simulink model "MISSILE_SIM_3DANIM"  (R2020b)
settings: Solver=ode4  StartTime=0.0  StopTime=45  FixedStep=0.01  RelTol=1e-3  EnableMultiTasking=on
undefined symbols (not defined in the file): d2r, Ka, Kdc, Ki, Kr, l_T0, V_T, X_M0, X_T0, Z_M0, Z_T0
libraries: vrlib x3, simulink x1
settings Model: Creator=vinay  LastModifiedBy=LeChinh
settings DataIOCC: LimitDataPoints=on  SaveFormat=Array  ReturnWorkspaceOutputs=off
settings OptimizationCC: LifeSpan=inf
settings DebuggingCC: SFUnexpectedBacktrackingDiag=warning  SFNoUnconditionalDefaultTransitionDiag=warning  SFExecutionAtInitializationDiag=none  ArithmeticOperatorsInVariantConditions=warning
settings HardwareCC: ProdBitPerPointer=32  ProdBitPerSizeT=32  ProdBitPerPtrDiffT=32  ProdLargestAtomicFloat=None  ProdIntDivRoundTo=Undefined  ProdEndianess=Unspecified  ProdWordSize=32  ProdHWDeviceType=32-bit Generic
settings ModelReferenceCC: PropagateSignalLabelsOutOfModel=off
settings SFSimCC: SimUseLocalCustomCode=off  CustomCodeUndefinedFunction=UseInterfaceOnly
settings RTWCC: RTWUseLocalCustomCode=off
settings CodeAppCC: StateflowObjectComments=on
settings GRTTargetCC: TargetLangStandard=C89/C90 (ANSI)
settings ConfigComp: CovMetricSettings=dw  CovSaveCumulativeToWorkspaceVar=on  CovSaveSingleToWorkspaceVar=on  CovExternalEMLEnable=off

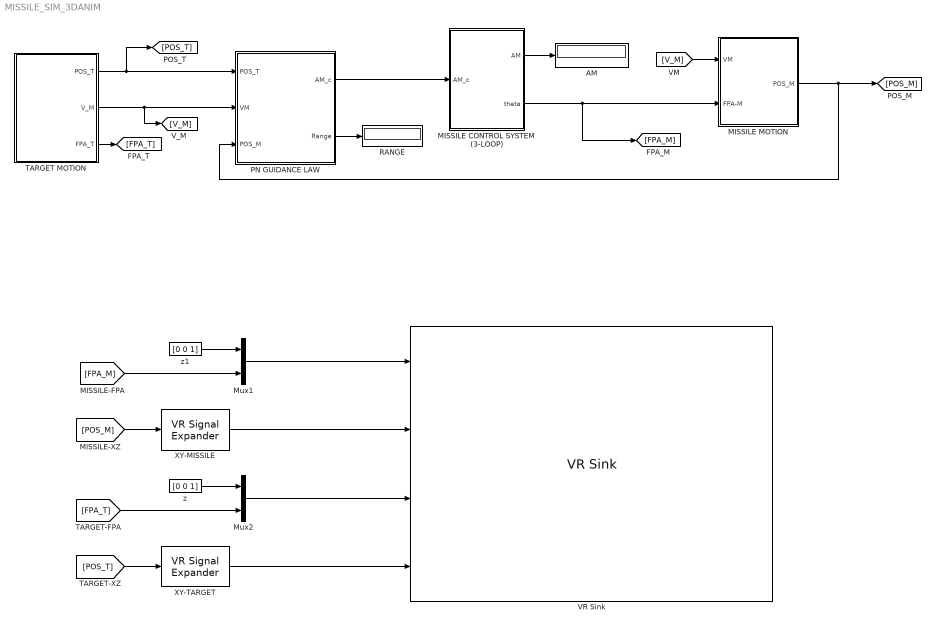
== system MISSILE_SIM_3DANIM ==
  AM : Display
  MISSILE CONTROL SYSTEM (3-LOOP) : Subsystem
  MISSILE MOTION : Subsystem
  Mux1 : Mux  Inputs=2
  Mux2 : Mux  Inputs=2
  PN GUIDANCE LAW : Subsystem
  RANGE : Display
  TARGET MOTION : Subsystem
  VR Sink : vrlib/VR Sink  InstantiateOnLoad=on  SampleTime=0.01  ViewEnable=on  RemoteChange=off  RemoteView=off  FieldsWritten=MISSILE-1_Scale.rotation.4.1.1.double#MISSILE-1_Scale.translation.3.1.1.double#UCAV_Halcyon_Test-3_Scale.rotation.4.1.1.double#UCAV_Halcyon_Test-3_Scale.translation.3.1.1.double  WorldFileName=interceptor_assembly.wrl  AutoView=off  VideoDimensions=[]  AllowVariableSize=off
  XY-MISSILE : vrlib/VR Signal Expander  outwidth=3  outidx=[1 2]
  XY-TARGET : vrlib/VR Signal Expander  outwidth=3  outidx=[1 2]
  z : Constant  Value=[0 0 1]
  z1 : Constant  Value=[0 0 1]
  wires:
  TARGET MOTION/1(POS_T) -> [POS_T], PN GUIDANCE LAW/1(POS_T)
  TARGET MOTION/2(V_M) -> [V_M], PN GUIDANCE LAW/2(VM)
  MISSILE MOTION/1(POS_M) -> PN GUIDANCE LAW/3(POS_M), [POS_M]
  MISSILE CONTROL SYSTEM (3-LOOP)/2(theta) -> [FPA_M], MISSILE MOTION/2(FPA-M)
  PN GUIDANCE LAW/1(AM_c) -> MISSILE CONTROL SYSTEM (3-LOOP)/1(AM_c)
  MISSILE CONTROL SYSTEM (3-LOOP)/1(AM) -> AM/1
  [V_M] -> MISSILE MOTION/1(VM)
  PN GUIDANCE LAW/2(Range) -> RANGE/1
  TARGET MOTION/3(FPA_T) -> [FPA_T]
  [POS_T] -> XY-TARGET/1
  [POS_M] -> XY-MISSILE/1
  [FPA_M] -> Mux1/2
  [FPA_T] -> Mux2/2
  z1/1 -> Mux1/1
  z/1 -> Mux2/1
  XY-MISSILE/1 -> VR Sink/2
  Mux2/1 -> VR Sink/3
  Mux1/1 -> VR Sink/1
  XY-TARGET/1 -> VR Sink/4

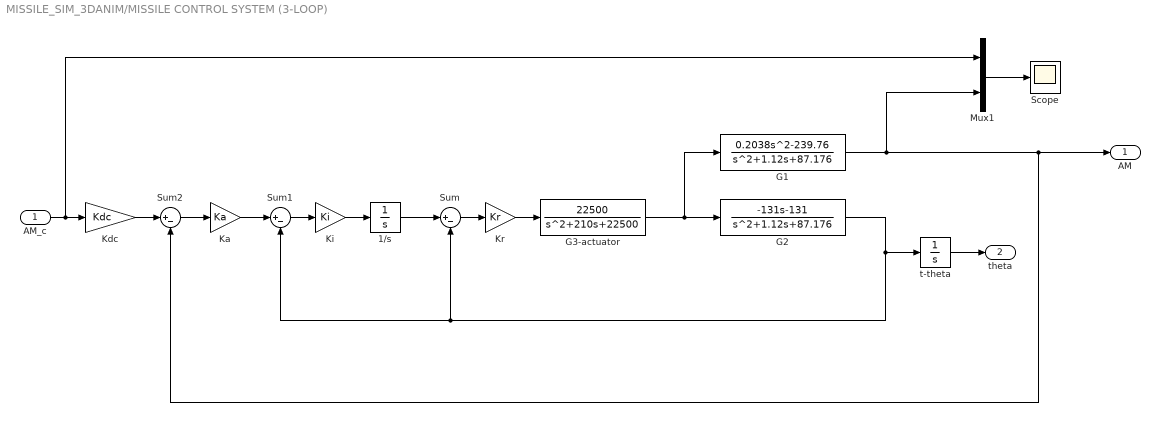
== system MISSILE_SIM_3DANIM/MISSILE CONTROL SYSTEM (3-LOOP) ==
  AM_c : Inport
  1/s : Integrator
  G1 : TransferFcn  Numerator=[0.2038, 0, -239.76]  Denominator=[1, 1.12, 87.176]
  G2 : TransferFcn  Numerator=[-131, -131]  Denominator=[1, 1.12, 87.176]
  G3-actuator : TransferFcn  Numerator=[22500]  Denominator=[1, 210, 22500]
  Ka : Gain  Gain=Ka
  Kdc : Gain  Gain=Kdc
  Ki : Gain  Gain=Ki
  Kr : Gain  Gain=Kr
  Mux1 : Mux  Inputs=2
  Scope : Scope
  Sum : Sum  Inputs=|+-
  Sum1 : Sum  Inputs=|+-
  Sum2 : Sum  Inputs=|+-
  t-theta : Integrator  InitialCondition=80*d2r
  AM : Outport
  theta : Outport  Port=2
  wires:
  Ki/1 -> 1/s/1
  Sum1/1 -> Ki/1
  t-theta/1 -> theta/1
  G3-actuator/1 -> G1/1, G2/1
  Kr/1 -> G3-actuator/1
  G2/1 -> t-theta/1, Sum1/2, Sum/2
  Sum/1 -> Kr/1
  1/s/1 -> Sum/1
  Ka/1 -> Sum1/1
  Kdc/1 -> Sum2/1
  Sum2/1 -> Ka/1
  AM_c/1 -> Mux1/1, Kdc/1
  G1/1 -> AM/1, Sum2/2, Mux1/2
  Mux1/1 -> Scope/1

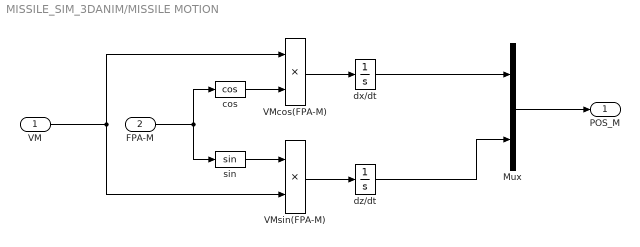
== system MISSILE_SIM_3DANIM/MISSILE MOTION ==
  VM : Inport
  FPA-M : Inport  Port=2
  Mux : Mux  Inputs=2
  VMcos(FPA-M) : Product
  VMsin(FPA-M) : Product
  cos : Trigonometry  Operator=cos
  dx/dt : Integrator  InitialCondition=X_M0
  dz/dt : Integrator  InitialCondition=Z_M0
  sin : Trigonometry
  POS_M : Outport
  wires:
  Mux/1 -> POS_M/1
  cos/1 -> VMcos(FPA-M)/2
  VMsin(FPA-M)/1 -> dz/dt/1
  sin/1 -> VMsin(FPA-M)/1
  VMcos(FPA-M)/1 -> dx/dt/1
  VM/1 -> VMsin(FPA-M)/2, VMcos(FPA-M)/1
  FPA-M/1 -> sin/1, cos/1
  dz/dt/1 -> Mux/2
  dx/dt/1 -> Mux/1

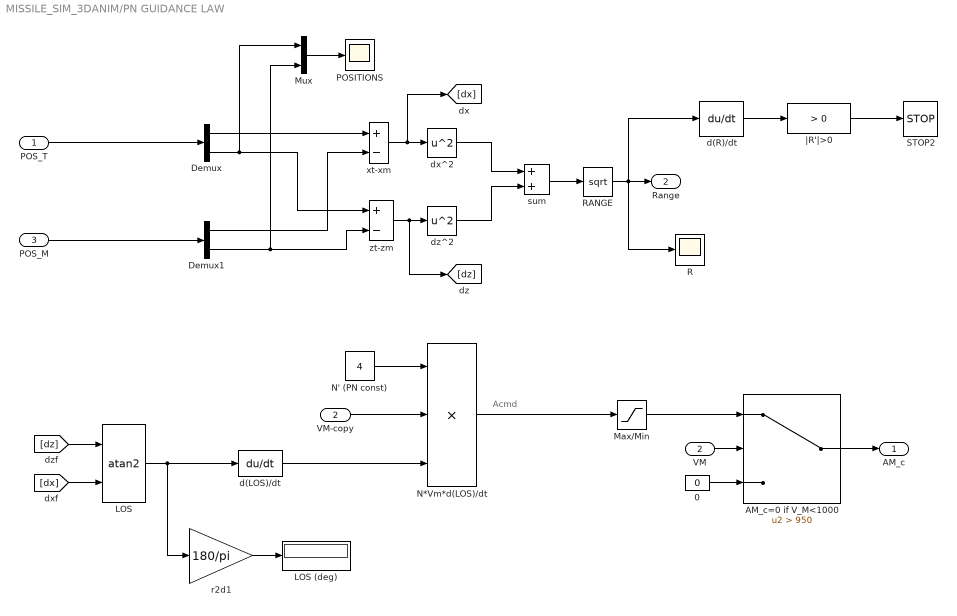
== system MISSILE_SIM_3DANIM/PN GUIDANCE LAW ==
  note: Acmd
  POS_T : Inport
  VM : Inport  Port=2
  POS_M : Inport  Port=3
  0 : Constant  Value=0
  AM_c=0 if V_M<1000 : Switch  Criteria=u2 > Threshold  Threshold=950
  Demux : Demux  Outputs=2
  Demux1 : Demux  Outputs=2
  LOS : Trigonometry  Operator=atan2  OutputSignalType=real
  LOS (deg) : Display
      settings: Format=bank
  Max/Min : Saturate  UpperLimit=0  LowerLimit=-0.10
  Mux : Mux  Inputs=2
  N' (PN const) : Constant  Value=4
  N*Vm*d(LOS)/dt : Product  Inputs=3
  POSITIONS : Scope
  R : Scope
  RANGE : Sqrt  OutputSignalType=real  SaturateOnIntegerOverflow=on
  STOP2 : Stop
  VM-copy : InportShadow  Port=2
  d(LOS)/dt : Derivative
  d(R)/dt : Derivative
  dx^2 : Math  Operator=square  SignedPower=on  OutputSignalType=real  SaturateOnIntegerOverflow=on
  dz^2 : Math  Operator=square  SignedPower=on  OutputSignalType=real  SaturateOnIntegerOverflow=on
  r2d1 : Gain  Gain=180/pi
  sum : Sum
  xt-xm : Sum  Inputs=+-
  zt-zm : Sum  Inputs=+-
  |R'|>0 : simulink/Logic and Bit Operations/Compare To Constant  relop=>  const=0  OutDataTypeStr=boolean
  AM_c : Outport
  Range : Outport  Port=2
  wires:
  AM_c=0 if V_M<1000/1 -> AM_c/1
  VM/1 -> AM_c=0 if V_M<1000/2
  POS_T/1 -> Demux/1
  POS_M/1 -> Demux1/1
  0/1 -> AM_c=0 if V_M<1000/3
  Demux/1 -> xt-xm/1
  Demux1/1 -> xt-xm/2
  Demux1/2 -> Mux/2, zt-zm/2
  Demux/2 -> Mux/1, zt-zm/1
  xt-xm/1 -> [dx], dx^2/1
  zt-zm/1 -> [dz], dz^2/1
  dx^2/1 -> sum/1
  dz^2/1 -> sum/2
  sum/1 -> RANGE/1
  RANGE/1 -> R/1, d(R)/dt/1, Range/1
  [dx] -> LOS/2
  LOS/1 -> d(LOS)/dt/1, r2d1/1
  d(LOS)/dt/1 -> N*Vm*d(LOS)/dt/3
  r2d1/1 -> LOS (deg)/1
  [dz] -> LOS/1
  N' (PN const)/1 -> N*Vm*d(LOS)/dt/1
  N*Vm*d(LOS)/dt/1 -> Max/Min/1
  VM-copy/1 -> N*Vm*d(LOS)/dt/2
  Max/Min/1 -> AM_c=0 if V_M<1000/1
  d(R)/dt/1 -> |R'|>0/1
  |R'|>0/1 -> STOP2/1
  Mux/1 -> POSITIONS/1

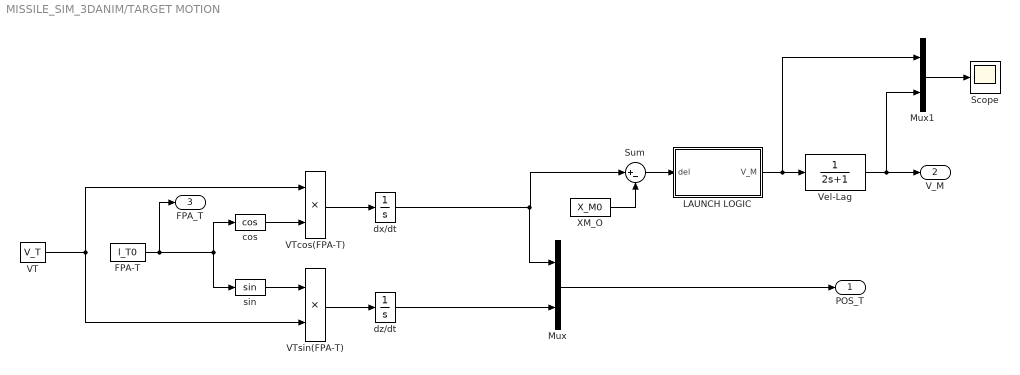
== system MISSILE_SIM_3DANIM/TARGET MOTION ==
  FPA-T : Constant  Value=l_T0
  LAUNCH LOGIC : MATLAB Function  TreatAsAtomicUnit=on
  Mux : Mux  Inputs=2
  Mux1 : Mux  Inputs=2
  Scope : Scope
  Sum : Sum  Inputs=|+-
  VT : Constant  Value=V_T
  VTcos(FPA-T) : Product
  VTsin(FPA-T) : Product
  Vel-Lag : TransferFcn  Denominator=[2 1]
  XM_O : Constant  Value=X_M0
  cos : Trigonometry  Operator=cos
  dx/dt : Integrator  InitialCondition=X_T0
  dz/dt : Integrator  InitialCondition=Z_T0
  sin : Trigonometry
  POS_T : Outport
  V_M : Outport  Port=2
  FPA_T : Outport  Port=3
  wires:
  cos/1 -> VTcos(FPA-T)/2
  LAUNCH LOGIC/1(V_M) -> Mux1/1, Vel-Lag/1
  dx/dt/1 -> Mux/1, Sum/1
  Sum/1 -> LAUNCH LOGIC/1(del)
  XM_O/1 -> Sum/2
  dz/dt/1 -> Mux/2
  Mux/1 -> POS_T/1
  VTsin(FPA-T)/1 -> dz/dt/1
  FPA-T/1 -> FPA_T/1, sin/1, cos/1
  VT/1 -> VTsin(FPA-T)/2, VTcos(FPA-T)/1
  sin/1 -> VTsin(FPA-T)/1
  VTcos(FPA-T)/1 -> dx/dt/1
  Vel-Lag/1 -> Mux1/2, V_M/1
  Mux1/1 -> Scope/1

== matlab function MISSILE_SIM_3DANIM/TARGET MOTION/LAUNCH LOGIC ==
  settings: updateMethod=DISCRETE
  data: del input; V_M output
function V_M = fcn(del)
%#codegen

persistent f
persistent Vel

if isempty(f)
    f = 0;
end
if isempty(Vel)
    Vel = 0;
end

if f == 0 && del > -200
    f = 1;
    Vel = 1021;
end


V_M = Vel;
